simulink model "sync_subsystem_example_org"  (Simulink 10.0)
settings: Solver=FixedStepDiscrete  StartTime=0.0  StopTime=10.0  RelTol=1e-3
libraries: hdlsllib x1, simulink x1
settings Model: DataTypeOverride=Off  Creator=cchung  LastModifiedBy=bhisma
settings Model: LogicAnalyzerGraphicalSettings=|
  | {
  |   "cursors" : {
  |     "activeCursor" : 0,
  |     "lockedCursors" : [
  | 
  |     ],
  |     "startingCursor" : 0,
  |     "times" : [
  |       0
  |     ]
  |   },
  |   "global" : {
  |     "fontSize" : 12,
  |     "height" : 14
  |   },
  |   "panels" : [
  |     {
  |       "height" : 100,
  |       "startingTrace" : 0,
  |       "traces" : [
  |         {
  |           "signalId" : "b6726206-d7c6-4cdc-ae89-adeec956ca08",
  |           "type" : "wave"
  |         },
  |         {
  |           "signalId" : "7b6508bf-70ac-40ed-89d1-cef4394d1f0a",
  |           "type" : "wave"
  |         },
  |         {
  |           "signalId" : "bdacf9d1-30ea-40bf-9fa7-345121fa2964",
  |           "type" : "wave"
  |         },
  |         {
  |           "signalId" : "96fa0b94-ce21-4eaf-9011-ad28c7263f2b",
  |           "type" : "wave"
  |         },
  |         {
  |           "signalId" : "f1342c8c-bf8e-43bd-9bb5-f8707e8cd8b4",
  |           "type" : "wave"
  |         }
  |       ],
  |       "yOffset" : 0
  |     }
  |   ],
  |   "timeAxis" : {
  |     "pixelsPerSecond" : 40.5
  |   }
  | }
settings DataIOCC: SaveFormat=Dataset  SaveOutput=off  SaveTime=off
settings OptimizationCC: BlockReduction=off  ConditionallyExecuteInputs=off  DefaultParameterBehavior=Inlined  LifeSpan=auto
settings DebuggingCC: AlgebraicLoopMsg=error  UnderspecifiedInitializationDetection=Simplified  MergeDetectMultiDrivingBlocksExec=error  SingleTaskRateTransMsg=error  StrictBusMsg=ErrorOnBusTreatedAsVector  SFUnexpectedBacktrackingDiag=error  SFNoUnconditionalDefaultTransitionDiag=error  SFExecutionAtInitializationDiag=warning
settings HardwareCC: ProdHWDeviceType=ASIC/FPGA->ASIC/FPGA  ProdEqTarget=off
settings ModelReferenceCC: PropagateSignalLabelsOutOfModel=on
settings GRTTargetCC: TargetLangStandard=C99 (ISO)  CombineOutputUpdateFcns=on  GRTInterface=off
settings ConfigComp: CovMetricSettings=dwe  CovHtmlReporting=off  CovSaveCumulativeToWorkspaceVar=off  CovSaveSingleToWorkspaceVar=off

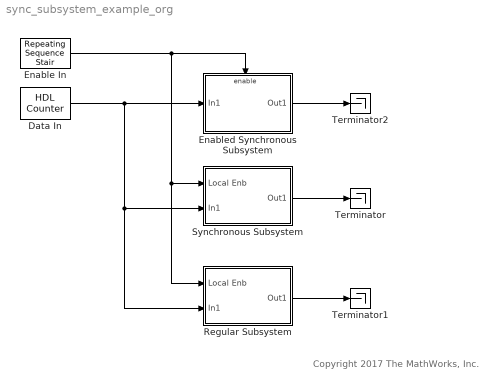
== system sync_subsystem_example_org ==
  note: Copyright 2017 The MathWorks, Inc.
  Data In : hdlsllib/Sources/HDL Counter  CountType=Free running  CountInit=0  CountStep=1  CountMax=25  CountFromType=Initial value  CountFrom=0  CountResetPort=off  CountLoadPort=off  CountEnbPort=off  CountDirPort=off  CountDataType=Unsigned  CountWordLen=8  CountFracLen=0  CountSampTime=1
      settings: SourceProductName=Simulink
  Enable In : simulink/Sources/Repeating Sequence Stair  OutValues=[0 1 0 0 1 1 0 0]  tsamp=1  OutMin=[]  OutMax=[]  OutDataTypeStr=fixdt('boolean')  OutputDataTypeScalingMode=Specify via dialog  OutDataType=fixdt('boolean')  ConRadixGroup=Best Precision: Vector-wise  OutScaling=[]
  Enabled Synchronous Subsystem : Subsystem  TreatAsAtomicUnit=on
  Regular Subsystem : Subsystem
  Synchronous Subsystem : Subsystem
  Terminator : Terminator
  Terminator1 : Terminator
  Terminator2 : Terminator
  wires:
  Data In/1 -> Regular Subsystem/2(In1), Synchronous Subsystem/2(In1), Enabled Synchronous Subsystem/1(In1)
  Synchronous Subsystem/1(Out1) -> Terminator/1
  Regular Subsystem/1(Out1) -> Terminator1/1
  Enable In/1 -> Regular Subsystem/1(Local Enb), Synchronous Subsystem/1(Local Enb), Enabled Synchronous Subsystem/Enable
  Enabled Synchronous Subsystem/1(Out1) -> Terminator2/1

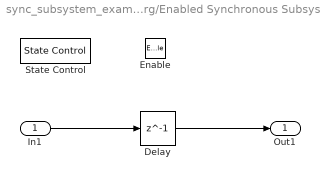
== system sync_subsystem_example_org/Enabled Synchronous Subsystem ==
  In1 : Inport
  Enable : EnablePort
  Delay : Delay  DelayLength=1
  State Control : StateControl  StateControl=Synchronous
  Out1 : Outport
  wires:
  In1/1 -> Delay/1
  Delay/1 -> Out1/1

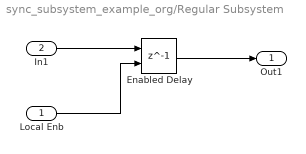
== system sync_subsystem_example_org/Regular Subsystem ==
  Local Enb : Inport
  In1 : Inport  Port=2
  Enabled Delay : Delay  DelayLength=1  ShowEnablePort=on
      settings: InputPortMap=u0,e6
  Out1 : Outport
  wires:
  In1/1 -> Enabled Delay/1
  Local Enb/1 -> Enabled Delay/2
  Enabled Delay/1 -> Out1/1

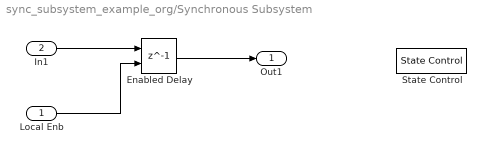
== system sync_subsystem_example_org/Synchronous Subsystem ==
  Local Enb : Inport
  In1 : Inport  Port=2
  Enabled Delay : Delay  DelayLength=1  ShowEnablePort=on
      settings: InputPortMap=u0,e6
  State Control : StateControl  StateControl=Synchronous
  Out1 : Outport
  wires:
  In1/1 -> Enabled Delay/1
  Local Enb/1 -> Enabled Delay/2
  Enabled Delay/1 -> Out1/1
